simulink model "linear_acceleration"  (R2024b)
settings: Solver=VariableStepAuto  StartTime=0.0  StopTime=10.0  RelTol=1e-3
settings Model: Creator=shohei  LastModifiedBy=shohei

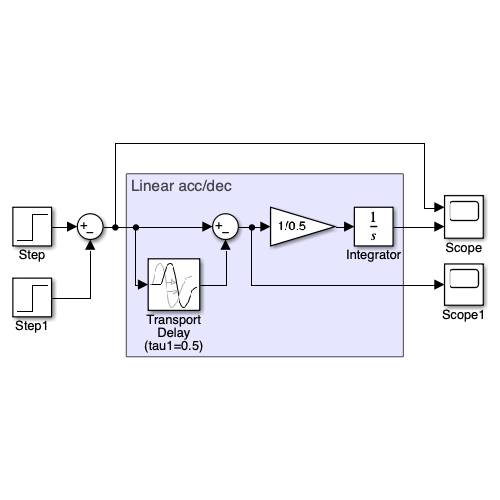
[thumbnail: Simulink's stored preview of the top-level diagram]
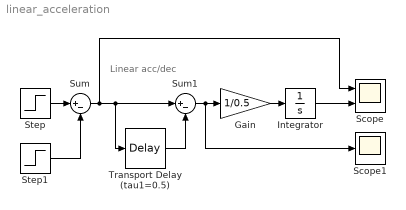
== system linear_acceleration ==
  note: Linear acc/dec
  Gain : Gain  Gain=1/0.5
  Integrator : Integrator
  Scope : Scope  NumInputPorts=2
  Scope1 : Scope
  Step : Step  SampleTime=0
  Step1 : Step  Time=4  SampleTime=0
  Sum : Sum  Inputs=|+-
  Sum1 : Sum  Inputs=|+-
  Transport Delay (tau1=0.5) : TransportDelay  DelayTime=0.5
  wires:
  Gain/1 -> Integrator/1
  Sum/1 -> Scope/1, Transport Delay (tau1=0.5)/1, Sum1/1
  Step1/1 -> Sum/2
  Step/1 -> Sum/1
  Sum1/1 -> Scope1/1, Gain/1
  Transport Delay (tau1=0.5)/1 -> Sum1/2
  Integrator/1 -> Scope/2
